simulink model "NoPedro"  (Simulink 7.9)
settings: Solver=ode45  StartTime=0.0  StopTime=10.0  RelTol=1e-3
settings Model: Creator=Administrator  LastModifiedBy=BLuu

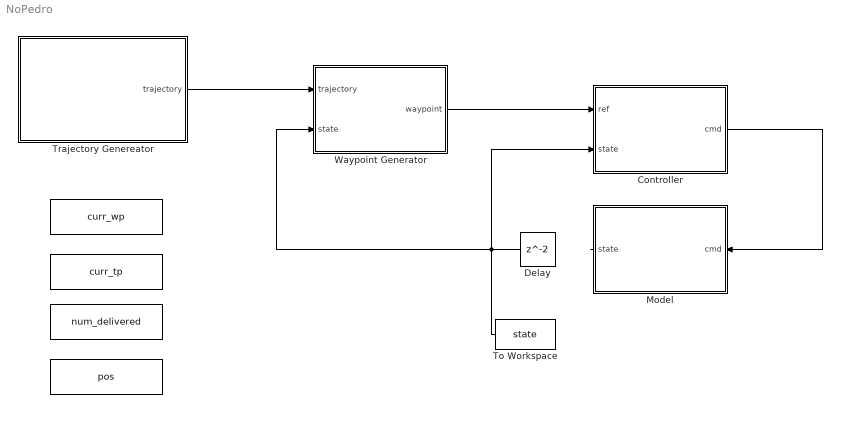
== system NoPedro ==
  " " : DataStoreMemory  DataStoreName=num_delivered  ReadBeforeWriteMsg=warning  WriteAfterWriteMsg=warning  WriteAfterReadMsg=warning  OutDataTypeStr=double
  "       " : DataStoreMemory  DataStoreName=curr_wp  ReadBeforeWriteMsg=warning  WriteAfterWriteMsg=warning  WriteAfterReadMsg=warning  OutDataTypeStr=double
  "         " : DataStoreMemory  DataStoreName=pos  ReadBeforeWriteMsg=warning  WriteAfterWriteMsg=warning  WriteAfterReadMsg=warning  InitialValue=[ 0 ; 0 ; 0 ]  OutDataTypeStr=double
  "          " : DataStoreMemory  DataStoreName=curr_tp  ReadBeforeWriteMsg=warning  WriteAfterWriteMsg=warning  WriteAfterReadMsg=warning  InitialValue=2  OutDataTypeStr=double
  Controller : MATLAB Function  TreatAsAtomicUnit=on
  Delay : Delay
  Model : MATLAB Function  TreatAsAtomicUnit=on
  To Workspace : ToWorkspace  VariableName=state  SampleTime=-1  SaveFormat=Structure With Time
  Trajectory Genereator : Subsystem
  Waypoint Generator : MATLAB Function  TreatAsAtomicUnit=on
  wires:
  Trajectory Genereator/1(trajectory) -> Waypoint Generator/1(trajectory)
  Controller/1(cmd) -> Model/1(cmd)
  Model/1(state) -> ?Integrator/1
  Waypoint Generator/1(waypoint) -> Controller/1(ref)
  Delay/1 -> To Workspace/1, Waypoint Generator/2(state), Controller/2(state)

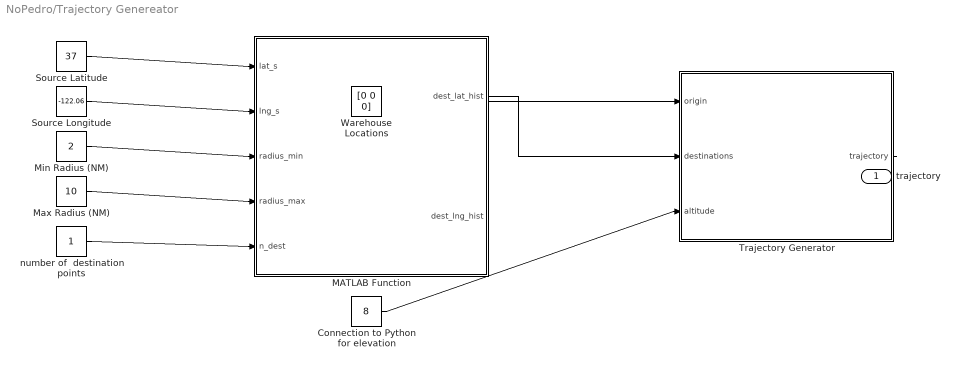
== system NoPedro/Trajectory Genereator ==
  Connection to Python for elevation : Constant  Value=8
  MATLAB Function : MATLAB Function  TreatAsAtomicUnit=on
  Max Radius (NM) : Constant  Value=10
  Min Radius (NM) : Constant  Value=2
  Source Latitude : Constant  Value=37
  Source Longitude : Constant  Value=-122.06
  Trajectory Generator : MATLAB Function  TreatAsAtomicUnit=on
  Warehouse Locations : Constant  Value=[0 0 0]
  number of  destination points : Constant
  trajectory : Outport
  wires:
  Warehouse Locations/1 -> Trajectory Generator/1(origin)
  Connection to Python for elevation/1 -> Trajectory Generator/3(altitude)
  MATLAB Function/1(dest_lat_hist) -> Trajectory Generator/2(destinations)
  Source Latitude/1 -> MATLAB Function/1(lat_s)
  Source Longitude/1 -> MATLAB Function/2(lng_s)
  Min Radius (NM)/1 -> MATLAB Function/3(radius_min)
  Max Radius (NM)/1 -> MATLAB Function/4(radius_max)
  number of  destination points/1 -> MATLAB Function/5(n_dest)
  Trajectory Generator/1(trajectory) -> trajectory/1

== matlab function Waypoint Generator ==
  data: trajectory input double; waypoint output double; state input double; curr_wp data_store_memory double; curr_tp data_store_memory double; num_delivered data_store_memory double
function waypoint = fcn(trajectory)
%#codegen
coder.extrinsic('display')
%display('current state:')
%state

global curr_wp curr_tp num_delivered pos;

% acceptable distance to waypoint
threshold = 1.5;

%% Trajectory Points
% origin      = trajectory(1,:);
% point1      = trajectory(2,:);
% point2      = trajectory(3,:);
% destination = trajectory(4,:);

%% Quadcopters current position
% if(length(state)== 1)
%     quad_X = 0;
%     quad_Y = 0;
%     quad_Z = 0;
% else
%     quad_X = state(1);
%     quad_Y = state(2);
%     quad_Z = state(3);
% end
quad_X = pos(1);
quad_Y = pos(2);
quad_Z = pos(3);
%% Specify last and next trajectory points
last_tp = trajectory(curr_tp - 1,:);
next_tp = trajectory(curr_tp,:);

%% Divide distance between last_wp and next_wp into evenly divided segments
% waypoint distances
wp_separation_dist = 1; 

% trajectory point distances
tp_separation_dist = sqrt((last_tp(1)-next_tp(1))^2 + (last_tp(2)-next_tp(2))^2 + (last_tp(3)-next_tp(3))^2);

%% Determine which segment to give next
number_of_waypoints = floor(tp_separation_dist/wp_separation_dist);
vec_norm = [(last_tp(1)-next_tp(1)) (last_tp(2)-next_tp(2)) (last_tp(3)-next_tp(3))]/tp_separation_dist;
if(isnan(vec_norm(1))) vec_norm(1) = 0; end
if(isnan(vec_norm(2))) vec_norm(2) = 0; end
if(isnan(vec_norm(3))) vec_norm(3) = 0; end
wp = last_tp + curr_wp*wp_separation_dist*-vec_norm;

% distance to current waypoint
dist1 = sqrt((quad_X-wp(1))^2 + (quad_Y-wp(2))^2 + (quad_Z-wp(3))^2);

if(dist1 <= threshold)
    curr_wp = curr_wp + 1;
    if(curr_wp == number_of_waypoints)
        curr_tp = curr_tp + 1;
        curr_wp = 0;
    end
end
if(curr_tp == length(trajectory(:,1)) + 1)
    curr_tp = 2;
    num_delivered = num_delivered + 1;
end

%p = zeros(15,1);
%p(1:3) = wp;

%% output
waypoint = wp;
end

== matlab function Trajectory Genereator/Trajectory Generator ==
  data: trajectory output double; origin input double; destinations input double; altitude input double; num_delivered data_store_memory double
function trajectory = fcn(origin,destinations, altitude)

%% Initialize variables
global num_delivered;
dest = [0 0 0];
trajectory = zeros(7,3);
origin = [0 0 0];
destinations = [10 10 0; 0 15 0; 10 15 0];

%% Set destination
destinations(:,1) = -destinations(:,1);
num_dest_points = length(destinations(:))/3;
if(num_dest_points > num_delivered)
    dest(1,:) = destinations(num_delivered+1,:);
end

waypoint1 = [origin(1) origin(2) -altitude];
waypoint2 = [dest(1,1) dest(1,2) -altitude];

trajectory = [origin ; waypoint1 ; waypoint2 ; dest ; waypoint2 ; waypoint1 ; origin];

== matlab function Trajectory Genereator/MATLAB Function ==
  data: lat_s input double; dest_lat_hist output double; lng_s input double; radius_min input double; radius_max input double; n_dest input double; dest_lng_hist output double
function [dest_lat_hist, dest_lng_hist] = dest_generator(lat_s, lng_s, radius_min, radius_max, n_dest)
%UNTITLED Summary of this function goes here
%   Detailed explanation goes here
% proc_simulate_destination
%

% lat_s = 37.0000; % Source latitude(degrees)
% lng_s = -122.0600; % Source longitude(degrees)
% radius_min = 2; % nautical-miles
% radius_max = 10; %nautical-miles
% n_dest = 10;
print_on = 0; % 0 turns it off. 1 turns it on
plot_on = 0;  % 0 turns it off. 1 turns it on
%

dest_lat_hist = 0;%zeros(n_dest,1);
dest_lng_hist = 0;%zeros(n_dest,1);
for i = 1:n_dest
    [lat,lng]=simulate_destination_v2(lat_s,lng_s,radius_min,radius_max);
    if (print_on == 1)
        fprintf('Latitude = %f (degrees) Longitude = %f (degrees)\n',lat, lng);
    end
    dest_lat_hist = lat;
    dest_lng_hist = lng;
end

if(plot_on)
    plot(dest_lng_hist,dest_lat_hist,'xb','MarkerSize',10);
    hold on;
    plot([lng_s,lng_s],[lat_s,lat_s],'or','MarkerSize',10);
    xlabel('Longitude (degrees)','FontSize',18);
    ylabel('Latitude (degrees)','FontSize',18);
    set(gca,'Fontsize',18,'LineWidth',2);
    grid on;
end

%dest = [dest_lat_hist, dest_lng_hist];

end

== matlab function Controller ==
  data: ref input double; cmd output double; curr_wp data_store_memory double; curr_tp data_store_memory double; num_delivered data_store_memory double; state input double; pos data_store_memory double
function cmd = Controller( ref , state)
% Controller for point-mass model of quadcopter
cmd = zeros(3,1);
global pos;

pos = state(1:3);
%ref = [1;1;0];
Ex = ref(1) - pos(1); % Error in x-direction
Ey = ref(2) - pos(2); % Error in y-direction
Ez = ref(3) - pos(3); % Error in z-direction

Xg = atan2(Ey,Ex);  % tracking angle

% 
% thresh = .25; % temporary threshold to see which way we are heading
% thresh_z = .25;
% 
% 
% Vg = 0;
% Vh = 0;
%  
% if( abs(Ex) >= thresh || abs(Ey) >= thresh )    % moving along x/y
%     Vg = 1;                                     % use ground speed
% end
% if ( Ez >= thresh_z && Ez ~= 0 )                   
%     Vh = Ez;                                 
% elseif ( Ez <= thresh_z && Ez ~= 0 )                   
%     Vh = Ez;              
% end

Vg = abs(Ex) + abs(Ey);
Vh = Ez;

cmd = [ Xg ; Vh ; Vg ];
end

== matlab function Model ==
  data: cmd
function state = Model( cmd )
% Point-mass model of quadcopter
state = zeros(3,1);

% Current position
global pos;
%cmd = [0.7854; 0; 1];
Xg = cmd(1); % tracking angle
Vh = cmd(2); % climb rate
Vg = cmd(3); % ground speed

x_dot = Vg*cos(Xg); % rate of change in x-direction
y_dot = Vg*sin(Xg); % rate of change in y-direction
z_dot = Vh;         % rate of change in z-direction

% state(1) = pos(1) + x_dot; % new x-pos
% state(2) = pos(2) + y_dot; % new y-pos
% state(3) = pos(3) + z_dot; % new z-pos
% pos = state;

state = [ x_dot ; y_dot ; z_dot ];
end
